simulink model "Lab2"  (R2022a)
settings: Solver=VariableStepAuto  StartTime=0.0  StopTime=3600  RelTol=1e-3
settings Model: Creator=이진진  LastModifiedBy=이진진
settings DebuggingCC: UnconnectedInputMsg=warning  UnconnectedOutputMsg=warning  UnconnectedLineMsg=warning
settings RTWCC: DLArmComputeVersion=19.05

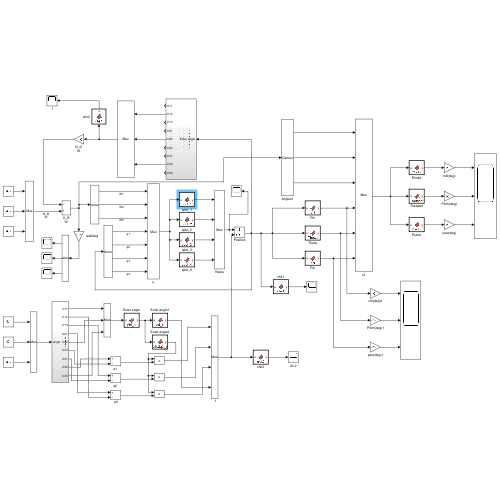
[thumbnail: Simulink's stored preview of the top-level diagram]
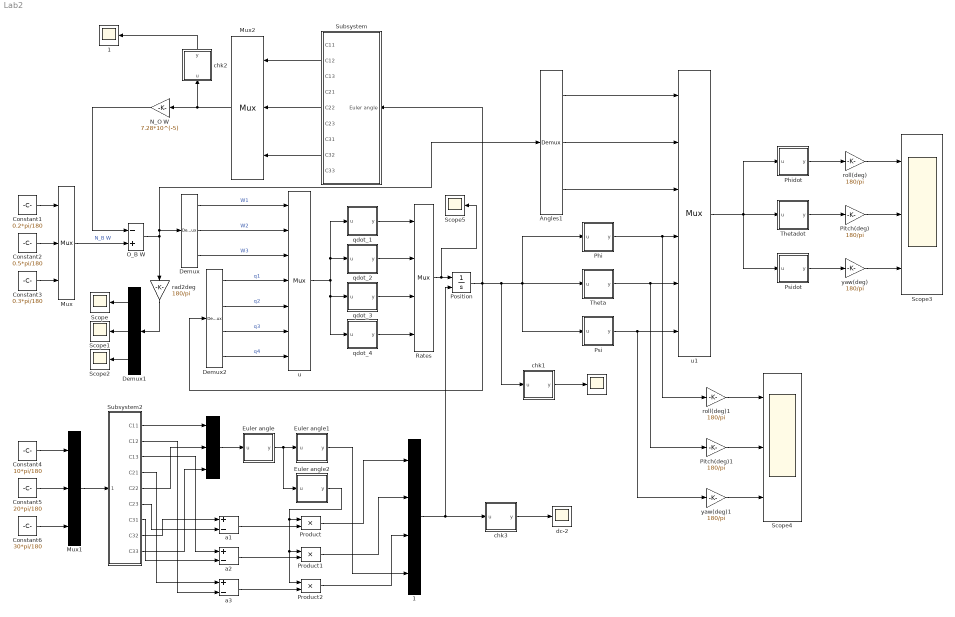
== system Lab2 ==
  " " : Scope
  "  " : Mux  Inputs=3
  "  1" : Mux
  " 1" : Scope
  " a2  " : Sum  Inputs=+-
  " a3" : Sum  Inputs=+-
  Angles1 : Demux  Outputs=3
      settings: DisplayOption=none
  Constant1 : Constant  Value=0.2*pi/180
  Constant2 : Constant  Value=0.5*pi/180
  Constant3 : Constant  Value=0.3*pi/180
  Constant4 : Constant  Value=10*pi/180
  Constant5 : Constant  Value=20*pi/180
  Constant6 : Constant  Value=30*pi/180
  Demux : Demux  Outputs=3
      settings: DisplayOption=none
  Demux1 : Demux  Outputs=3
      settings: DisplayOption=none
  Demux2 : Demux
      settings: DisplayOption=none
  Euler angle : MATLAB Function  TreatAsAtomicUnit=on
  Euler angle1 : MATLAB Function  TreatAsAtomicUnit=on
  Euler angle2 : MATLAB Function  TreatAsAtomicUnit=on
  Mux : Mux  Inputs=3
  Mux1 : Mux  Inputs=3
  Mux2 : Mux  Inputs=3
  N_O W : Gain  Gain=7.28*10^(-5)
  O_B W : Sum  Inputs=-+
  Phi : MATLAB Function  TreatAsAtomicUnit=on
  Phidot : MATLAB Function  TreatAsAtomicUnit=on
  Pitch(deg) : Gain  Gain=180/pi
  Pitch(deg)1 : Gain  Gain=180/pi
  Position : Integrator  InitialConditionSource=external  InitialCondition=[10*pi/180, 20*pi/180, 30*pi/180]
  Product : Product
  Product1 : Product
  Product2 : Product
  Psi : MATLAB Function  TreatAsAtomicUnit=on
  Psidot : MATLAB Function  TreatAsAtomicUnit=on
  Rates : Mux
  Scope{,1..2,5} (4 alike) : Scope
  Scope3 : Scope  NumInputPorts=3
  Scope4 : Scope  NumInputPorts=3
  Subsystem : Subsystem
  Subsystem2 : Subsystem
  Theta : MATLAB Function  TreatAsAtomicUnit=on
  Thetadot : MATLAB Function  TreatAsAtomicUnit=on
  "a1 " : Sum  Inputs=+-
  chk1 : MATLAB Function  TreatAsAtomicUnit=on
  chk2 : MATLAB Function  TreatAsAtomicUnit=on
  chk3 : MATLAB Function  TreatAsAtomicUnit=on
  dc-2 : Scope
  qdot_1 : MATLAB Function  TreatAsAtomicUnit=on
  qdot_2 : MATLAB Function  TreatAsAtomicUnit=on
  qdot_3 : MATLAB Function  TreatAsAtomicUnit=on
  qdot_4 : MATLAB Function  TreatAsAtomicUnit=on
  rad2deg : Gain  Gain=180/pi
  roll(deg) : Gain  Gain=180/pi
  roll(deg)1 : Gain  Gain=180/pi
  u : Mux  Inputs=7
  u1 : Mux  Inputs=6
  yaw(deg) : Gain  Gain=180/pi
  yaw(deg)1 : Gain  Gain=180/pi
  wires:
  Demux/1 -> u/1  "W1"
  Demux/2 -> u/2  "W2"
  Demux/3 -> u/3  "W3"
  Demux1/1 -> Scope/1
  Demux1/2 -> Scope1/1
  Demux1/3 -> Scope2/1
  Demux2/1 -> u/4  "q1"
  Demux2/2 -> u/5  "q2"
  Demux2/3 -> u/6  "q3"
  Constant1/1 -> Mux/1
  Constant2/1 -> Mux/2
  Constant3/1 -> Mux/3
  Mux/1 -> O_B W/2  "N_B W"
  O_B W/1 -> Angles1/1, Demux/1, rad2deg/1
  u/1 -> qdot_4/1(u), qdot_3/1(u), qdot_2/1(u), qdot_1/1(u)
  qdot_1/1(y) -> Rates/1
  qdot_2/1(y) -> Rates/2
  qdot_3/1(y) -> Rates/3
  Rates/1 -> Scope5/1, Position/1
  Phidot/1(y) -> roll(deg)/1
  Thetadot/1(y) -> Pitch(deg)/1
  Psidot/1(y) -> yaw(deg)/1
  Pitch(deg)/1 -> Scope3/2
  yaw(deg)/1 -> Scope3/3
  Subsystem/2(C12) -> Mux2/1
  Subsystem/5(C22) -> Mux2/2
  Subsystem/8(C32) -> Mux2/3
  Mux2/1 -> chk2/1(u), N_O W/1
  N_O W/1 -> O_B W/1
  chk1/1(y) -> " "/1
  Demux2/4 -> u/7  "q4"
  qdot_4/1(y) -> Rates/4
  Position/1 -> Demux2/1, Subsystem/1(Euler angle), Psi/1(u), Phi/1(u), Theta/1(u), chk1/1(u)
  chk2/1(y) -> " 1"/1
  Phi/1(y) -> roll(deg)1/1, u1/4
  Theta/1(y) -> Pitch(deg)1/1, u1/5
  Psi/1(y) -> yaw(deg)1/1, u1/6
  Angles1/1 -> u1/1
  Angles1/2 -> u1/2
  Angles1/3 -> u1/3
  u1/1 -> Psidot/1(u), Phidot/1(u), Thetadot/1(u)
  roll(deg)1/1 -> Scope4/1
  Pitch(deg)1/1 -> Scope4/2
  yaw(deg)1/1 -> Scope4/3
  Constant4/1 -> Mux1/1
  Constant5/1 -> Mux1/2
  Constant6/1 -> Mux1/3
  Mux1/1 -> Subsystem2/1(angle)
  Subsystem2/1(C11) -> "  "/1
  Subsystem2/5(C22) -> "  "/2
  Subsystem2/9(C33) -> "  "/3
  "  "/1 -> Euler angle/1(u)
  Euler angle/1(y) -> Euler angle2/1(u), Euler angle1/1(u)
  Subsystem2/8(C32) -> "a1 "/1
  Subsystem2/6(C23) -> "a1 "/2
  Subsystem2/3(C13) -> " a2  "/1
  Subsystem2/7(C31) -> " a2  "/2
  Subsystem2/4(C21) -> " a3"/1
  Subsystem2/2(C12) -> " a3"/2
  "a1 "/1 -> Product/2
  " a2  "/1 -> Product1/2
  " a3"/1 -> Product2/2
  Euler angle2/1(y) -> Product/1, Product1/1, Product2/1
  Product/1 -> "  1"/1
  Product1/1 -> "  1"/2
  Product2/1 -> "  1"/3
  Euler angle1/1(y) -> "  1"/4
  "  1"/1 -> Position/2, chk3/1(u)
  chk3/1(y) -> dc-2/1
  rad2deg/1 -> Demux1/1
  roll(deg)/1 -> Scope3/1

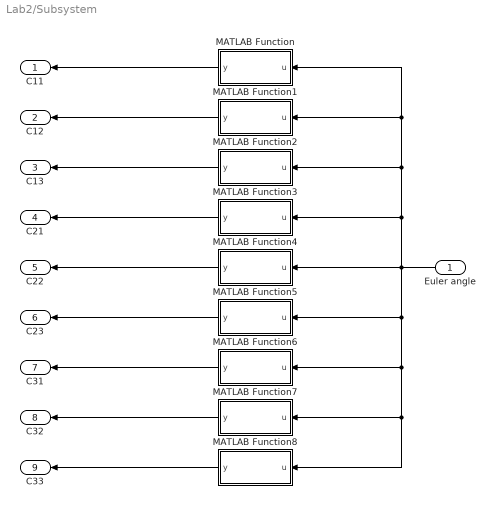
== system Lab2/Subsystem ==
  Euler angle : Inport
  MATLAB Function : MATLAB Function  TreatAsAtomicUnit=on
  MATLAB Function1 : MATLAB Function  TreatAsAtomicUnit=on
  MATLAB Function2 : MATLAB Function  TreatAsAtomicUnit=on
  MATLAB Function3 : MATLAB Function  TreatAsAtomicUnit=on
  MATLAB Function4 : MATLAB Function  TreatAsAtomicUnit=on
  MATLAB Function5 : MATLAB Function  TreatAsAtomicUnit=on
  MATLAB Function6 : MATLAB Function  TreatAsAtomicUnit=on
  MATLAB Function7 : MATLAB Function  TreatAsAtomicUnit=on
  MATLAB Function8 : MATLAB Function  TreatAsAtomicUnit=on
  C11 : Outport
  C12 : Outport  Port=2
  C13 : Outport  Port=3
  C21 : Outport  Port=4
  C22 : Outport  Port=5
  C23 : Outport  Port=6
  C31 : Outport  Port=7
  C32 : Outport  Port=8
  C33 : Outport  Port=9
  wires:
  MATLAB Function8/1(y) -> C33/1
  MATLAB Function7/1(y) -> C32/1
  MATLAB Function6/1(y) -> C31/1
  MATLAB Function5/1(y) -> C23/1
  MATLAB Function4/1(y) -> C22/1
  MATLAB Function3/1(y) -> C21/1
  MATLAB Function2/1(y) -> C13/1
  MATLAB Function1/1(y) -> C12/1
  MATLAB Function/1(y) -> C11/1
  Euler angle/1 -> MATLAB Function/1(u), MATLAB Function1/1(u), MATLAB Function2/1(u), MATLAB Function3/1(u), MATLAB Function4/1(u), MATLAB Function5/1(u), MATLAB Function6/1(u), MATLAB Function7/1(u), MATLAB Function8/1(u)

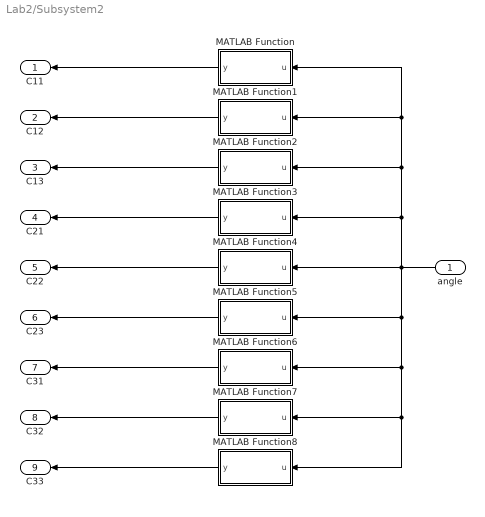
== system Lab2/Subsystem2 ==
  angle : Inport
  MATLAB Function : MATLAB Function  TreatAsAtomicUnit=on
  MATLAB Function1 : MATLAB Function  TreatAsAtomicUnit=on
  MATLAB Function2 : MATLAB Function  TreatAsAtomicUnit=on
  MATLAB Function3 : MATLAB Function  TreatAsAtomicUnit=on
  MATLAB Function4 : MATLAB Function  TreatAsAtomicUnit=on
  MATLAB Function5 : MATLAB Function  TreatAsAtomicUnit=on
  MATLAB Function6 : MATLAB Function  TreatAsAtomicUnit=on
  MATLAB Function7 : MATLAB Function  TreatAsAtomicUnit=on
  MATLAB Function8 : MATLAB Function  TreatAsAtomicUnit=on
  C11 : Outport
  C12 : Outport  Port=2
  C13 : Outport  Port=3
  C21 : Outport  Port=4
  C22 : Outport  Port=5
  C23 : Outport  Port=6
  C31 : Outport  Port=7
  C32 : Outport  Port=8
  C33 : Outport  Port=9
  wires:
  MATLAB Function8/1(y) -> C33/1
  MATLAB Function7/1(y) -> C32/1
  MATLAB Function6/1(y) -> C31/1
  MATLAB Function5/1(y) -> C23/1
  MATLAB Function4/1(y) -> C22/1
  MATLAB Function3/1(y) -> C21/1
  MATLAB Function2/1(y) -> C13/1
  MATLAB Function1/1(y) -> C12/1
  MATLAB Function/1(y) -> C11/1
  angle/1 -> MATLAB Function/1(u), MATLAB Function1/1(u), MATLAB Function2/1(u), MATLAB Function3/1(u), MATLAB Function4/1(u), MATLAB Function5/1(u), MATLAB Function6/1(u), MATLAB Function7/1(u), MATLAB Function8/1(u)

== matlab function Lab2/qdot_2 ==
  data: u input; y output
function y = qdot_2(u)

y = (1/2)*(-u(3)*u(4) + u(1)*u(6) + u(2)*u(7))

end

== matlab function Lab2/qdot_4 ==
  data: u input; y output
function y = qdot_4(u)

y = (1/2)*(-u(1)*u(4) - u(2)*u(5) - u(3)*u(6));

end

== matlab function Lab2/chk2 ==
  data: u input; y output
function y = chk1(u)

y = u(1)^2 + u(2)^2 + u(3)^2;

end

== matlab function Lab2/Phi ==
  data: u input; y output
function y = phi(u)

y = atan(2*(u(1)*u(4) + u(2)*u(3))/(1-2*(u(1)^2 + u(2)^2)));

end

== matlab function Lab2/Theta ==
  data: u input; y output
function y = Thetat(u)

y = asin(2*(u(2)*u(4) - u(3)*u(1)));

end

== matlab function Lab2/Psi ==
  data: u input; y output
function y = psi(u)

y = atan((2*(u(3)*u(4) + u(1)*u(2)))/(1-2*(u(2)^2+u(3)^2)));

end

== matlab function Lab2/Phidot ==
  data: u input; y output
function y = Phidot(u)

y = u(1) + sin(u(4))*tan(u(5))*u(2) + cos(u(4))*tan(u(5))*u(3);

end

== matlab function Lab2/Thetadot ==
  data: u input; y output
function y = Thetadot(u)

y = cos(u(4))*u(2) - sin(u(4))*u(3);

end

== matlab function Lab2/Psidot ==
  data: u input; y output
function y = Psidot(u)

y = (sin(u(4))/cos(u(5)))*u(2) + (cos(u(4))/cos(u(5))*u(3));

end

== matlab function Lab2/Euler angle ==
  data: y output; u input
function y = phi_p(u)

y = acos((u(1) + u(2) + u(3) - 1) / 2);

end

== matlab function Lab2/Euler angle1 ==
  data: y output; u input
function y = q4_e(u)

y = cos(u/2);

end

== matlab function Lab2/qdot_1 ==
  data: u input; y output
function y = qdot_1(u)

y = (1/2)*(u(3)*u(5) - u(2)*u(6) + u(1)*u(7));

end

== matlab function Lab2/Euler angle2 ==
  data: y output; u input
function y = q1q2q3_e(u)

y = 1/(4*cos(u/2));

end

== matlab function Lab2/chk3 ==
  data: u input; y output
function y = chk2(u)

y = u(1)^2 + u(2)^2 + u(3)^2 + u(4)^2;

end

== matlab function Lab2/Subsystem2/MATLAB Function ==
  data: u input; y output
function y = C11(u)

y = cos(u(3))*cos(u(2));

end

== matlab function Lab2/Subsystem2/MATLAB Function1 ==
  data: u input; y output
function y = C12(u)

y = sin(u(3))*cos(u(2));

end

== matlab function Lab2/Subsystem2/MATLAB Function2 ==
  data: u input; y output
function y = C13(u)

y = -sin(u(2));

end

== matlab function Lab2/Subsystem2/MATLAB Function3 ==
  data: u input; y output
function y = C21(u)

y = -sin(u(3))*cos(u(1)) + cos(u(3))*sin(u(2))*sin(u(1));

end

== matlab function Lab2/Subsystem2/MATLAB Function4 ==
  data: u input; y output
function y = C22(u)

y = cos(u(3))*cos(u(1)) + sin(u(3))*sin(u(2))*sin(u(1));

end

== matlab function Lab2/Subsystem2/MATLAB Function5 ==
  data: u input; y output
function y = C23(u)

y = cos(u(2))*sin(u(1));

end

== matlab function Lab2/Subsystem2/MATLAB Function6 ==
  data: u input; y output
function y = C31(u)

y = sin(u(3))*sin(u(1)) + cos(u(3))*sin(u(2))*cos(u(1));

end

== matlab function Lab2/Subsystem2/MATLAB Function7 ==
  data: u input; y output
function y = C32(u)

y = -cos(u(3))*sin(u(1)) + sin(u(3))*sin(u(2))*cos(u(1));

end

== matlab function Lab2/qdot_3 ==
  data: u input; y output
function y = qdot_3(u)

y = (1/2)*(u(2)*u(4) - u(1)*u(5) + u(3)*u(7));

end

== matlab function Lab2/Subsystem2/MATLAB Function8 ==
  data: u input; y output
function y = C33(u)

y = cos(u(2))*cos(u(1));

end

== matlab function Lab2/Subsystem/MATLAB Function ==
  data: u input; y output
function y = C11(u)

y = (u(1)^2 - u(2)^2 - u(3)^2 + u(4)^2);

end

== matlab function Lab2/Subsystem/MATLAB Function1 ==
  data: u input; y output
function y = C12(u)

y = 2*(u(1)*u(2) + u(3)*u(4));

end

== matlab function Lab2/Subsystem/MATLAB Function2 ==
  data: u input; y output
function y = C13(u)

y = 2*(u(1)*u(3) - u(2)*u(4));

end

== matlab function Lab2/Subsystem/MATLAB Function3 ==
  data: u input; y output
function y = C21(u)

y = 2*(u(1)*u(2) - u(3)*u(4));

end

== matlab function Lab2/Subsystem/MATLAB Function4 ==
  data: u input; y output
function y = C22(u)

y = (-u(1)^2 + u(2)^2 - u(3)^2 + u(4)^2);

end

== matlab function Lab2/Subsystem/MATLAB Function5 ==
  data: u input; y output
function y = C23(u)

y = 2*(u(2)*u(3) + u(1)*u(4));

end

== matlab function Lab2/Subsystem/MATLAB Function6 ==
  data: u input; y output
function y = C31(u)

y = 2*(u(1)*u(3) + u(2)*u(4));

end

== matlab function Lab2/Subsystem/MATLAB Function7 ==
  data: u input; y output
function y = C32(u)

y = 2*(u(2)*u(3) - u(1)*u(4));

end

== matlab function Lab2/Subsystem/MATLAB Function8 ==
  data: u input; y output
function y = C33(u)

y = 2*(-u(1)^2 - u(2)^2 + u(3)^2 + u(4)^2);

end

== matlab function Lab2/chk1 ==
  data: u input; y output
function y = chk1(u)

y = (u(1)^2 + u(2)^2 + u(3)^2 + u(4)^2);

end
